simulink model "Ex7_Validation_StateEstimation"  (R2025b)
settings: Solver=VariableStepAuto  StartTime=0.0  StopTime=60  RelTol=1e-3
undefined symbols (not defined in the file): anglerate, motor_param, PosEnc, VelEnc
libraries: simulink x3, sm_lib x3, SigiLib x3, slpidlib x1, robotcorelib x1, mspfiltlib x1, dspstat3 x1, nesl_utility x1
settings Model: Creator=resjoehr  LastModifiedBy=resjoehr

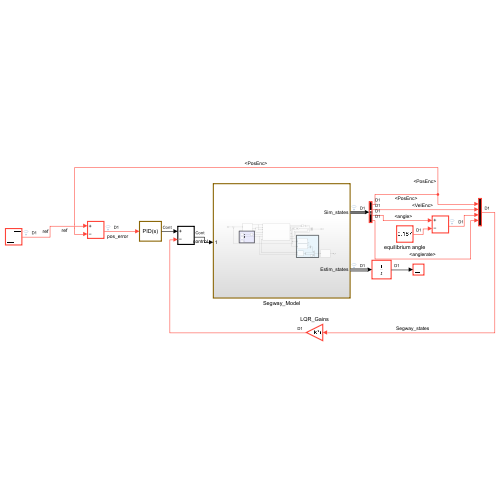
[thumbnail: Simulink's stored preview of the top-level diagram]
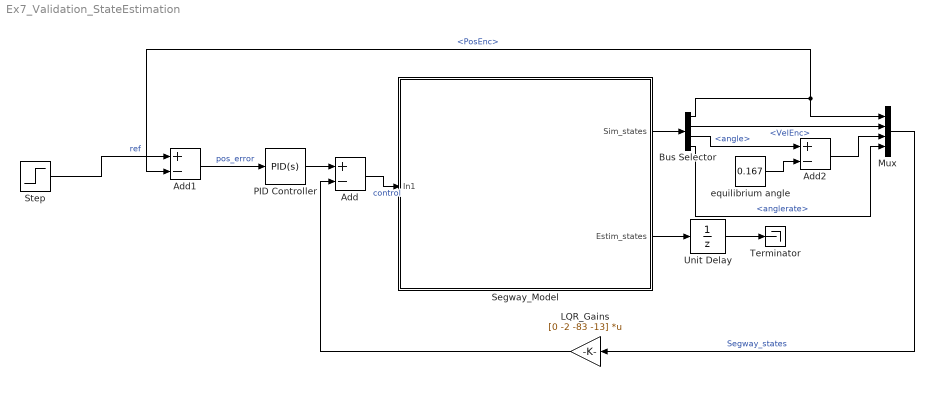
== system Ex7_Validation_StateEstimation ==
  Add : Sum  Inputs=+-
  Add1 : Sum  Inputs=+-
  Add2 : Sum  Inputs=+-
  Bus Selector : BusSelector  OutputSignals=PosEnc,VelEnc,angle,anglerate
  LQR_Gains : Gain  Gain=[0 -2 -83 -13]  Multiplication=Matrix(K*u)
  Mux : Mux
  PID Controller : slpidlib/PID Controller  Controller=PID  Form=Parallel  TimeDomain=Continuous-time  UseExternalTs=off  SampleTime=-1  IntegratorMethod=Forward Euler  FilterMethod=Forward Euler  ControllerParametersSource=internal  P=-1  I=0  UseKiTs=off  D=0  UseExternalDerivativeSource=off  N=100  UseFilter=on  TunerSelectOption=Transfer Function Based (PID Tuner App)  InitialConditionSource=internal  InitialConditionForIntegrator=0  InitialConditionForFilter=0  DifferentiatorICPrevScaledInput=0  ExternalReset=none  TrackingMode=off  Kt=1  LimitOutput=off  SatLimitsSource=internal  UpperSaturationLimit=inf  LowerSaturationLimit=-inf  LinearizeAsGain=on  AntiWindupMode=none  Kb=1  LimitIntegrator=off  UpperIntegratorSaturationLimit=inf  LowerIntegratorSaturationLimit=-inf  POutMin=[]  POutMax=[]  IOutMin=[]  IOutMax=[]  DOutMin=[]  DOutMax=[]  NOutMin=[]  NOutMax=[]  SumOutMin=[]  SumOutMax=[]  SaturationOutMin=[]  SaturationOutMax=[]  PParamMin=[]  PParamMax=[]  IParamMin=[]  IParamMax=[]  DParamMin=[]  DParamMax=[]  NParamMin=[]  NParamMax=[]  KbParamMin=[]  KbParamMax=[]  KtParamMin=[]  KtParamMax=[]  KbOutMin=[]  KbOutMax=[]  KtOutMin=[]  KtOutMax=[]  IntegratorOutMin=[]  IntegratorOutMax=[]  FilterOutMin=[]  FilterOutMax=[]  SumI1OutMin=[]  SumI1OutMax=[]  SumI2OutMin=[]  SumI2OutMax=[]  SumI3OutMin=[]  SumI3OutMax=[]  SumI4OutMin=[]  SumI4OutMax=[]  SumDOutMin=[]  SumDOutMax=[]  DifferentiatorOutMin=[]  DifferentiatorOutMax=[]  FilterDiffOutCoefMin=[]  FilterDiffOutCoefMax=[]  ReciprocalOutMin=[]  ReciprocalOutMax=[]  SumDenOutMin=[]  SumDenOutMax=[]  SumNumOutMin=[]  SumNumOutMax=[]  DivideOutMin=[]  DivideOutMax=[]  UdiffTsProdOutMin=[]  UdiffTsProdOutMax=[]  NTsProdOutMin=[]  NTsProdOutMax=[]  UintegralTsProdOutMin=[]  UintegralTsProdOutMax=[]  UngainTsProdOutMin=[]  UngainTsProdOutMax=[]  ClampingZeroOutDataTypeStr=Inherit: Inherit via back propagation  ClampingZeroOutMin=[]  ClampingZeroOutMax=[]  FilterDenConstantOutDataTypeStr=Inherit: Inherit via back propagation  FilterDenConstantOutMin=[]  FilterDenConstantOutMax=[]  PCopyOutDataTypeStr=Inherit: Inherit via back propagation  PCopyOutMin=[]  PCopyOutMax=[]  NCopyOutDataTypeStr=Inherit: Inherit via back propagation  NCopyOutMin=[]  NCopyOutMax=[]  IntegratorContinuousStateAttributes=''  IntegratorStateMustResolveToSignalObject=off  IntegratorRTWStateStorageClass=Auto  FilterContinuousStateAttributes=''  FilterStateMustResolveToSignalObject=off  FilterRTWStateStorageClass=Auto  ParallelPVariant=InternalParameters  IdealPVariant=Disabled  IVariant=InternalParameters  DVariant=InternalParameters  IntegratorVariant=Continuous  SatVariant=Disabled  AWVariant=Passthrough  PCopyVariant=Disabled  TRVariant=Disabled  FdbkBlocksVariant=Forward  IdealPFdbkVariant=Disabled  SatFdbkVariant=Disabled  DerivativeFilterVariant=ContFilter  NVariant=InternalParameters  NCopyVariant=Disabled  FilterICVariant=InternalICsFilter  IntegratorICVariant=InternalICs  ExternalResetVariant=Disabled  TRSumVariant=Passthrough  SumFdbkVariant=Disabled  SumVariant=Sum_PID  TsampFilterVariant=InternalTs  TsampNgainVariant=Passthrough  TsampIntegralVariant=Disabled_SignalSpec  ExternalSaturationOutDataTypeStr=Inherit: Same as second input  DerivativeSourceVariant=ErrorSignal  PreIntVariant=InternalPreInt
  Segway_Model : Subsystem
  Step : Step  Time=5  SampleTime=0.01
  Terminator : Terminator
  Unit Delay : UnitDelay  SampleTime=-1  HasFrameUpgradeWarning=on
  equilibrium angle : Constant  Value=0.167  SampleTime=0.01
  wires:
  Bus Selector/1 -> Mux/1, Add1/2  "<PosEnc>"
  Bus Selector/2 -> Mux/2  "<VelEnc>"
  Bus Selector/3 -> Add2/1  "<angle>"
  Bus Selector/4 -> Mux/4  "<anglerate>"
  Mux/1 -> LQR_Gains/1  "Segway_states"
  LQR_Gains/1 -> Add/2
  Add/1 -> Segway_Model/1(In1)  "control"
  Add2/1 -> Mux/3
  equilibrium angle/1 -> Add2/2
  Add1/1 -> PID Controller/1  "pos_error"
  PID Controller/1 -> Add/1
  Segway_Model/1(Sim_states) -> Bus Selector/1
  Segway_Model/2(Estim_states) -> Unit Delay/1
  Step/1 -> Add1/1  "ref"
  Unit Delay/1 -> Terminator/1

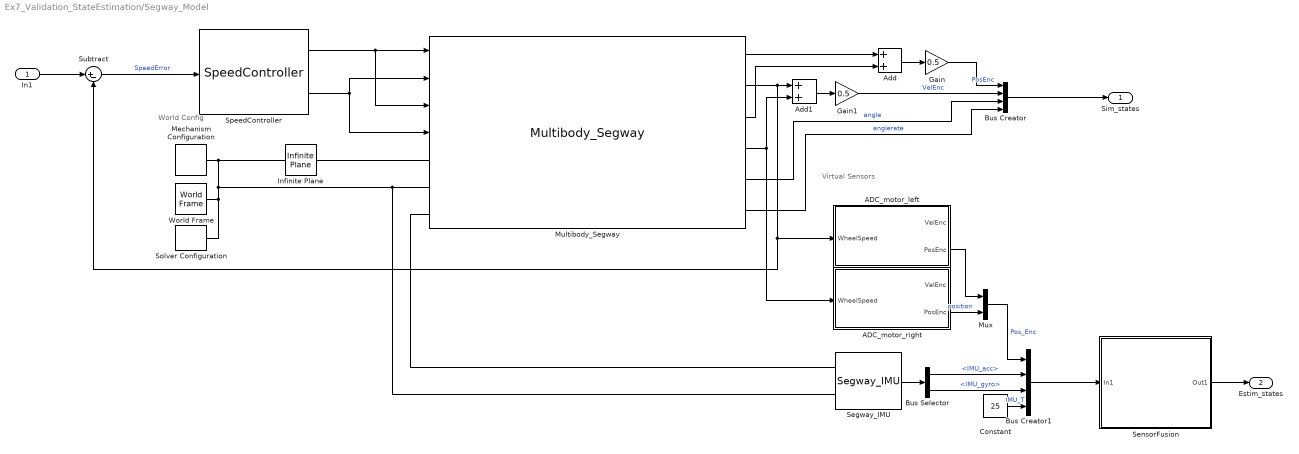
== system Ex7_Validation_StateEstimation/Segway_Model ==
  note: World Config
  note: Virtual Sensors
  In1 : Inport
  ADC_motor_left : Subsystem
  ADC_motor_right : Subsystem
  Add : Sum
  Add1 : Sum
  Bus Creator : BusCreator  Inputs=4  OutDataTypeStr=Bus: States
  Bus Creator1 : BusCreator  Inputs=4  OutDataTypeStr=Bus: Sensors
      settings: InheritFromInputs=off
  Bus Selector : BusSelector  OutputSignals=IMU_acc,IMU_gyro
  Constant : Constant  Value=25  SampleTime=0.01
  Gain : Gain  Gain=0.5
  Gain1 : Gain  Gain=0.5
  Infinite Plane : sm_lib/Curves and Surfaces/Infinite Plane  GraphicType=Rectangle  GraphicPlaneWidth=1  GraphicPlaneWidthUnits=m  GraphicPlaneHeight=1  GraphicPlaneHeightUnits=m  GraphicVisPropType=SimpleVisualProperties  GraphicDiffuseColor=[0.5 0.5 0.5]  GraphicOpacity=0.25  GraphicSpecularColor=[0.5 0.5 0.5 1.0]  GraphicAmbientColor=[0.15 0.15 0.15 1.0]  GraphicEmissiveColor=[0.0 0.0 0.0 1.0]  GraphicShininess=75
  Mechanism Configuration : sm_lib/Utilities/Mechanism Configuration  UniformGravity=Constant  GravityVector=[0 0 -9.80665]  GravityVectorUnits=m/s^2  LinearizationDelta=0.001  JointModeTransitionNonlinearIterations=2
  Multibody_Segway : SigiLib/Multibody_Segway  Parameter3=motor_left  Parameter2=motor_left
  Mux : Mux  Inputs=2
  Segway_IMU : SigiLib/Segway_IMU  SystemSampleTime=-1  VariantActivationTime=update diagram  EmptyChoice=off  PassThrough=off  PassThroughVariantControl=(default)  EmptyChoiceVariantControl=(default)  AllowFlexibleInterface=on  Latency=0  AutoFrameSizeCalculation=off
  SensorFusion : Subsystem
  Solver Configuration : nesl_utility/Solver Configuration  PhysicalDomain=network_engine_domain  SubClassName=solver  LeftPortType=input  RightPortType=generic  Tones=[]  Harmonics=[]  SimulateNoise=off  Profile=off  UseLocalSampling=off  EnableSwitchedLinearOptims=on  FrequencyDomain=off  UseCCode=off  RelTol=0.001  AbsTol=1e-06  MinStep=1e-09  ToWorkspace=off  RevertToSquareIcSolve=off  NumHomotopyIterations=100  PhasorMode=off  PhasorModeNumHarmonics=1  ConsistencySolver=NEWTON_FTOL  IndexReductionMethod=DerivativeReplacement  DoDC=off  ResidualTolerance=1e-09  ConsistencyTolSource=GLOBAL  ConsistencyAbsTol=0.001  ConsistencyRelTol=0.001  ConsistencyTolFactor=0.001  UseLocalSolver=off  LocalSolverChoice=NE_BACKWARD_EULER_ADVANCER  ResolveIndetEquations=on  FunctionEvalNumThread=1  LocalSolverSampleTime=0.001  DoFixedCost=off  MaxNonlinIter=3  MaxModeIter=2  ComputeImpulses=off  ImpulseIterations=2  LinearAlgebra=Sparse  LinearAlgebraNumThread=0  EquationFormulation=NE_TIME_EF  DelaysMemoryBudget=1024  AutomaticFiltering=on  FilteringTimeConstant=0.001  PartitionStorageMethod=AS_NEEDED  PartitionMemoryBudget=1024  PartitionMethod=FAST  MultibodyUseLocalSolver=off  MultibodyLocalSolverChoice=ODE1  MultibodyLocalSolverSampleTime=0.001
  SpeedController : SigiLib/SpeedController  p_gain=motor_left.P  i_gain=motor_left.I  d_gain=motor_left.D  n_filter=motor_left.N  direction=0
  Subtract : Sum  Inputs=|+-
  World Frame : sm_lib/Frames and Transforms/World Frame
  Sim_states : Outport
  Estim_states : Outport  Port=2
  wires:
  In1/1 -> Subtract/1
  Subtract/1 -> SpeedController/1  "SpeedError"
  SpeedController/1 -> Multibody_Segway/3, Multibody_Segway/1
  SpeedController/2 -> Multibody_Segway/4, Multibody_Segway/2
  Multibody_Segway/3 -> Add/2
  Multibody_Segway/1 -> Add/1
  ADC_motor_right/2(PosEnc) -> Mux/2  "position"
  Multibody_Segway/2 -> Add1/1, Subtract/2, ADC_motor_left/1(WheelSpeed)
  ADC_motor_left/2(PosEnc) -> Mux/1
  Mux/1 -> Bus Creator1/1  "Pos_Enc"
  Segway_IMU/1 -> Bus Selector/1
  Multibody_Segway/4 -> ADC_motor_right/1(WheelSpeed), Add1/2
  Bus Selector/2 -> Bus Creator1/3  "<IMU_gyro>"
  Constant/1 -> Bus Creator1/4  "IMU_T"
  Bus Creator1/1 -> SensorFusion/1(In1)
  Bus Selector/1 -> Bus Creator1/2  "<IMU_acc>"
  SensorFusion/1(Out1) -> Estim_states/1
  Add/1 -> Gain/1
  Gain/1 -> Bus Creator/1  "PosEnc"
  Add1/1 -> Gain1/1
  Gain1/1 -> Bus Creator/2  "VelEnc"
  Multibody_Segway/5 -> Bus Creator/3  "angle"
  Multibody_Segway/6 -> Bus Creator/4  "anglerate"
  Bus Creator/1 -> Sim_states/1
  connections:
  Infinite Plane/RConn1 -- Multibody_Segway/LConn1
  Segway_IMU/LConn2 -- Multibody_Segway/LConn2 -- World Frame/RConn1 -- Solver Configuration/RConn1 -- Infinite Plane/LConn1 -- Mechanism Configuration/RConn1
  Segway_IMU/LConn1 -- Multibody_Segway/LConn3

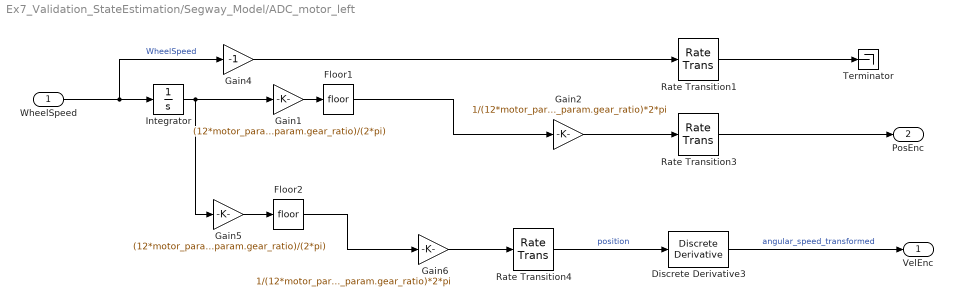
== system Ex7_Validation_StateEstimation/Segway_Model/ADC_motor_left ==
  WheelSpeed : Inport
  Discrete Derivative3 : simulink/Discrete/Discrete Derivative  gainval=1  ICPrevScaledInput=0.0  OutMin=[]  OutMax=[]  OutDataType=fixdt(1, 16)  OutScaling=2^-10  DoSatur=off
  Floor1 : Rounding
  Floor2 : Rounding
  Gain1 : Gain  Gain=(12*motor_param.motor_ratio*motor_param.gear_ratio)/(2*pi)
  Gain2 : Gain  Gain=1/(12*motor_param.motor_ratio*motor_param.gear_ratio)*2*pi  OutDataTypeStr=double
  Gain4 : Gain  Gain=-1
  Gain5 : Gain  Gain=(12*motor_param.motor_ratio*motor_param.gear_ratio)/(2*pi)
  Gain6 : Gain  Gain=1/(12*motor_param.motor_ratio*motor_param.gear_ratio)*2*pi  OutDataTypeStr=double
  Integrator : Integrator
  Rate Transition1 : RateTransition  OutPortSampleTime=0.01
  Rate Transition3 : RateTransition  OutPortSampleTime=0.01
  Rate Transition4 : RateTransition  OutPortSampleTime=0.01
  Terminator : Terminator
  VelEnc : Outport
  PosEnc : Outport  Port=2
  wires:
  WheelSpeed/1 -> Integrator/1, Gain4/1  "WheelSpeed"
  Rate Transition3/1 -> PosEnc/1
  Gain2/1 -> Rate Transition3/1
  Floor1/1 -> Gain2/1
  Integrator/1 -> Gain5/1, Gain1/1
  Rate Transition1/1 -> Terminator/1
  Gain4/1 -> Rate Transition1/1
  Discrete Derivative3/1 -> VelEnc/1  "angular_speed_transformed"
  Gain1/1 -> Floor1/1
  Gain5/1 -> Floor2/1
  Floor2/1 -> Gain6/1
  Gain6/1 -> Rate Transition4/1
  Rate Transition4/1 -> Discrete Derivative3/1  "position"

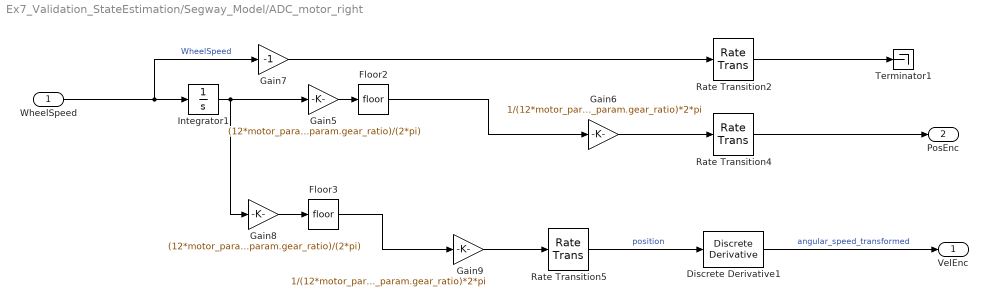
== system Ex7_Validation_StateEstimation/Segway_Model/ADC_motor_right ==
  WheelSpeed : Inport
  Discrete Derivative1 : simulink/Discrete/Discrete Derivative  gainval=1  ICPrevScaledInput=0.0  OutMin=[]  OutMax=[]  OutDataType=fixdt(1, 16)  OutScaling=2^-10  DoSatur=off
  Floor2 : Rounding
  Floor3 : Rounding
  Gain5 : Gain  Gain=(12*motor_param.motor_ratio*motor_param.gear_ratio)/(2*pi)
  Gain6 : Gain  Gain=1/(12*motor_param.motor_ratio*motor_param.gear_ratio)*2*pi  OutDataTypeStr=double
  Gain7 : Gain  Gain=-1
  Gain8 : Gain  Gain=(12*motor_param.motor_ratio*motor_param.gear_ratio)/(2*pi)
  Gain9 : Gain  Gain=1/(12*motor_param.motor_ratio*motor_param.gear_ratio)*2*pi  OutDataTypeStr=double
  Integrator1 : Integrator
  Rate Transition2 : RateTransition  OutPortSampleTime=0.01
  Rate Transition4 : RateTransition  OutPortSampleTime=0.01
  Rate Transition5 : RateTransition  OutPortSampleTime=0.01
  Terminator1 : Terminator
  VelEnc : Outport
  PosEnc : Outport  Port=2
  wires:
  Rate Transition2/1 -> Terminator1/1
  Gain9/1 -> Rate Transition5/1
  Floor3/1 -> Gain9/1
  Rate Transition5/1 -> Discrete Derivative1/1  "position"
  Floor2/1 -> Gain6/1
  Rate Transition4/1 -> PosEnc/1
  Gain7/1 -> Rate Transition2/1
  Integrator1/1 -> Gain8/1, Gain5/1
  WheelSpeed/1 -> Integrator1/1, Gain7/1  "WheelSpeed"
  Gain5/1 -> Floor2/1
  Gain8/1 -> Floor3/1
  Discrete Derivative1/1 -> VelEnc/1  "angular_speed_transformed"
  Gain6/1 -> Rate Transition4/1

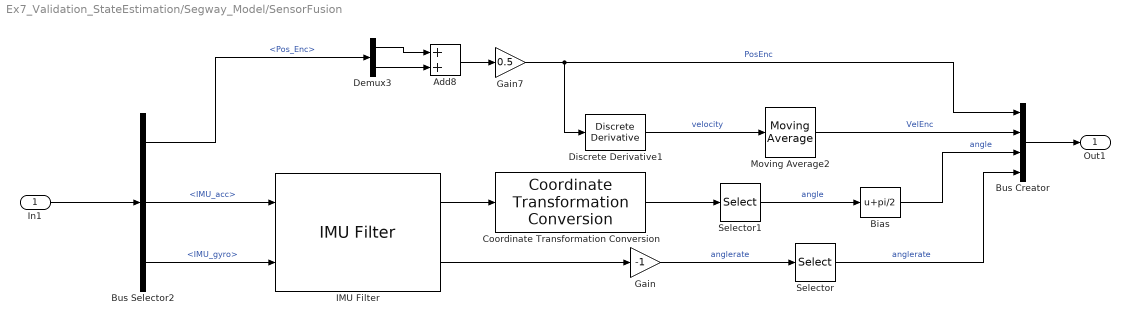
== system Ex7_Validation_StateEstimation/Segway_Model/SensorFusion ==
  In1 : Inport
  Add8 : Sum
  Bias : Bias  Bias=pi/2  SaturateOnIntegerOverflow=off
  Bus Creator : BusCreator  Inputs=PosEnc,VelEnc,angle,anglerate  OutDataTypeStr=Bus: States
  Bus Selector2 : BusSelector  OutputSignals=Pos_Enc,IMU_acc,IMU_gyro
  Coordinate Transformation Conversion : robotcorelib/Coordinate Transformation Conversion  InputRepresentation=Rotation Matrix  InputEulerSequence=ZYX  ShowTrVecInputPort=on  OutputRepresentation=Euler Angles  OutputEulerSequence=XYZ  ShowTrVecOutputPort=on  SimulateUsing=Interpreted execution
      settings: LibrarySourceBlock=navlib/Utilities/Coordinate Transformation Conversion
  Demux3 : Demux  Outputs=2
  Discrete Derivative1 : simulink/Discrete/Discrete Derivative  gainval=1.0  ICPrevScaledInput=0.0  OutMin=[]  OutMax=[]  OutDataType=fixdt(1, 16)  OutScaling=2^-10  DoSatur=off
  Gain : Gain  Gain=-1
  Gain7 : Gain  Gain=0.5
  IMU Filter : mspfiltlib/IMU Filter  DispRefFrame=NED  OrientationFormat=Rotation matrix  DecimationFactor=1  InitialProcessNoise=imufilter.defaultProcessNoise  AccelerometerNoise=2.2693e-4  GyroscopeNoise=2.4065e-5  GyroscopeDriftNoise=3.0462e-13  LinearAccelerationNoise=0.0096236100000000012  LinearAccelerationDecayFactor=0.5  SimulateUsing=Interpreted execution
  Moving Average2 : dspstat3/Moving Average  Method=Sliding window  ForgettingFactorPort=off  SpecifyWindowLength=on  WindowLength=4  OverlapLength=3  AllowArbitraryInputLength=off  ForgettingFactor=0.9  SimulateUsing=Interpreted execution
  Selector : Selector  InputPortWidth=3  IndexOptions=Index vector (dialog)  Indices=[1]  OutputSizes=1
  Selector1 : Selector  InputPortWidth=3  IndexOptions=Index vector (dialog)  Indices=[1]  OutputSizes=1
  Out1 : Outport  OutDataTypeStr=Bus: States
  wires:
  Gain7/1 -> Bus Creator/1, Discrete Derivative1/1  "PosEnc"
  Demux3/2 -> Add8/2
  Discrete Derivative1/1 -> Moving Average2/1  "velocity"
  Bus Selector2/1 -> Demux3/1  "<Pos_Enc>"
  IMU Filter/1 -> Coordinate Transformation Conversion/1
  IMU Filter/2 -> Gain/1
  Bus Selector2/2 -> IMU Filter/1  "<IMU_acc>"
  Add8/1 -> Gain7/1
  Selector1/1 -> Bias/1  "angle"
  Bus Selector2/3 -> IMU Filter/2  "<IMU_gyro>"
  Demux3/1 -> Add8/1
  Coordinate Transformation Conversion/1 -> Selector1/1
  Selector/1 -> Bus Creator/4  "anglerate"
  Bus Creator/1 -> Out1/1
  In1/1 -> Bus Selector2/1
  Moving Average2/1 -> Bus Creator/2  "VelEnc"
  Bias/1 -> Bus Creator/3  "angle"
  Gain/1 -> Selector/1  "anglerate"
